simulink model "Tank_Overflow_Prevention"  (R2020a)
settings: Solver=FixedStepAuto  StartTime=0.0  StopTime=inf  FixedStep=0.002  RelTol=1e-3  EnableMultiTasking=on
libraries: simulink_extras x2
settings Model: ExtModeTrigDuration=10000  Creator=therobo956  LastModifiedBy=orlando.cobos
settings SolverCC: PositivePriorityOrder=on
settings DataIOCC: ReturnWorkspaceOutputs=off
settings DebuggingCC: PregeneratedLibrarySubsystemCodeDiagnostic=none  ArithmeticOperatorsInVariantConditions=warning
settings SFSimCC: SimUseLocalCustomCode=off  CustomCodeUndefinedFunction=UseInterfaceOnly
settings RTWCC: Description=QUARC Win64 Target  SystemTargetFile=quarc_win64.tlc  TemplateMakefile=quarc_default_tmf  RTWUseLocalCustomCode=off
settings STFCustomTargetCC: TargetPreCompLibLocation=C:\PROGRA~3\QUARC\lib\2019a\win64\release  TargetLangStandard=C99 (ISO)  ConcurrentExecutionCompliant=on  GRTInterface=on  SystemTargetFile=quarc_win64.tlc
settings GRTTargetCC: TargetPreCompLibLocation=C:\PROGRA~3\QUARC\lib\2019a\win64\release  ParMdlRefBuildCompliant=off  CompOptLevelCompliant=off  CombineOutputUpdateFcns=off  MatFileLogging=off  CPPClassGenCompliant=off  GRTInterface=on  UseToolchainInfoCompliant=off  ExtMode=on  ExtModeMexFile=quarc_comm

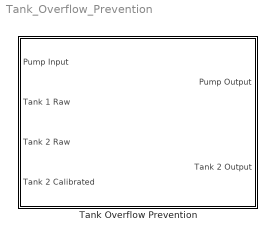
== system Tank_Overflow_Prevention ==
  Tank Overflow Prevention : Subsystem

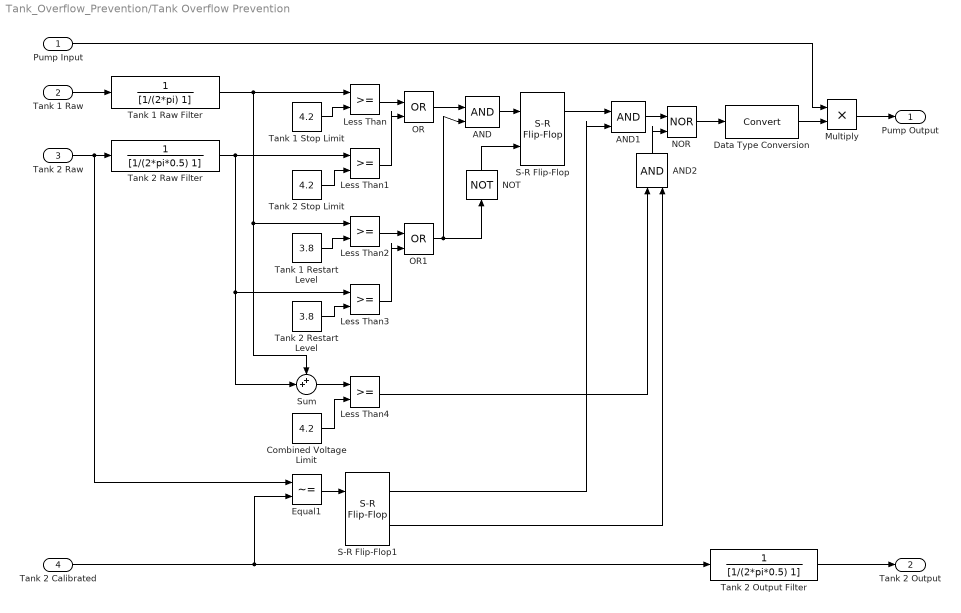
== system Tank_Overflow_Prevention/Tank Overflow Prevention ==
  Pump Input : Inport
  Tank 1 Raw : Inport  Port=2
  Tank 2 Raw : Inport  Port=3
  Tank 2 Calibrated : Inport  Port=4
  AND : Logic  IconShape=distinctive  AllPortsSameDT=off  OutDataTypeStr=boolean
  AND1 : Logic  IconShape=distinctive  AllPortsSameDT=off  OutDataTypeStr=boolean
  AND2 : Logic  IconShape=distinctive  AllPortsSameDT=off  OutDataTypeStr=boolean
  Combined Voltage Limit : Constant  Value=4.2
  Data Type Conversion : DataTypeConversion  OutMin=[0]  OutMax=[1]
  Equal1 : RelationalOperator  Operator=~=  OutDataTypeStr=boolean  RndMeth=Simplest
  Less Than{,1..4} (5 alike) : RelationalOperator  RndMeth=Simplest
  Multiply : Product
  NOR : Logic  Operator=NOR  IconShape=distinctive  AllPortsSameDT=off  OutDataTypeStr=boolean
  NOT : Logic  Operator=NOT  IconShape=distinctive  AllPortsSameDT=off  OutDataTypeStr=boolean
  OR : Logic  Operator=OR  IconShape=distinctive  AllPortsSameDT=off  OutDataTypeStr=boolean
  OR1 : Logic  Operator=OR  IconShape=distinctive  AllPortsSameDT=off  OutDataTypeStr=boolean
  S-R Flip-Flop : simulink_extras/Flip Flops/S-R Flip-Flop  initial_condition=0
  S-R Flip-Flop1 : simulink_extras/Flip Flops/S-R Flip-Flop  initial_condition=0
  Sum : Sum  Inputs=++|
  Tank 1 Raw Filter : TransferFcn  Denominator=[1/(2*pi) 1]
  Tank 1 Restart Level : Constant  Value=3.8
  Tank 1 Stop Limit : Constant  Value=4.2
  Tank 2 Output Filter : TransferFcn  Denominator=[1/(2*pi*0.5) 1]
  Tank 2 Raw Filter : TransferFcn  Denominator=[1/(2*pi*0.5) 1]
  Tank 2 Restart Level : Constant  Value=3.8
  Tank 2 Stop Limit : Constant  Value=4.2
  Pump Output : Outport  VectorParamsAs1DForOutWhenUnconnected=off
  Tank 2 Output : Outport  Port=2  VectorParamsAs1DForOutWhenUnconnected=off
  wires:
  Multiply/1 -> Pump Output/1
  Pump Input/1 -> Multiply/1
  Tank 1 Stop Limit/1 -> Less Than/2
  Tank 2 Stop Limit/1 -> Less Than1/2
  Less Than/1 -> OR/1
  Less Than1/1 -> OR/2
  Data Type Conversion/1 -> Multiply/2
  Tank 1 Restart Level/1 -> Less Than2/2
  Tank 2 Restart Level/1 -> Less Than3/2
  Less Than2/1 -> OR1/1
  Less Than3/1 -> OR1/2
  OR/1 -> AND/1
  OR1/1 -> AND/2, NOT/1
  AND/1 -> S-R Flip-Flop/1
  NOT/1 -> S-R Flip-Flop/2
  Sum/1 -> Less Than4/1
  Combined Voltage Limit/1 -> Less Than4/2
  Less Than4/1 -> AND2/1
  NOR/1 -> Data Type Conversion/1
  AND2/1 -> NOR/2
  S-R Flip-Flop/1 -> AND1/1
  AND1/1 -> NOR/1
  S-R Flip-Flop1/1 -> AND1/2
  Tank 2 Calibrated/1 -> Equal1/2, Tank 2 Output Filter/1
  S-R Flip-Flop1/2 -> AND2/2
  Equal1/1 -> S-R Flip-Flop1/1
  Tank 2 Output Filter/1 -> Tank 2 Output/1
  Tank 1 Raw Filter/1 -> Sum/1, Less Than2/1, Less Than/1
  Tank 2 Raw/1 -> Tank 2 Raw Filter/1, Equal1/1
  Tank 2 Raw Filter/1 -> Sum/2, Less Than3/1, Less Than1/1
  Tank 1 Raw/1 -> Tank 1 Raw Filter/1
